simulink library "lib_FOWLTY"  (R2022a)
settings: Solver=ode45  StartTime=0.0  StopTime=10.0  RelTol=1e-3  EnableMultiTasking=on
undefined symbols (not defined in the file or in its folder): sigbuilder_block, tMax, wind
libraries: simulink x1
settings Model: Creator=grunnet  LastModifiedBy=Yerai
settings SolverCC: AlgebraicLoopSolver=TrustRegion
settings DataIOCC: LimitDataPoints=on  SaveFormat=Array  ReturnWorkspaceOutputs=off
settings OptimizationCC: ExpressionDepthLimit=2147483647  LifeSpan=inf
settings DebuggingCC: UnderspecifiedInitializationDetection=Classic  MergeDetectMultiDrivingBlocksExec=none  SolverPrmCheckMsg=warning  FcnCallInpInsideContextMsg=warning  UnconnectedInputMsg=warning  UnconnectedOutputMsg=warning  UnconnectedLineMsg=warning  StateNameClashWarn=warning  SFUnexpectedBacktrackingDiag=warning  SFNoUnconditionalDefaultTransitionDiag=warning  SFExecutionAtInitializationDiag=none  ArithmeticOperatorsInVariantConditions=warning
settings HardwareCC: ProdBitPerPointer=32  ProdBitPerSizeT=32  ProdBitPerPtrDiffT=32  ProdLargestAtomicFloat=None  ProdIntDivRoundTo=Undefined  ProdEndianess=Unspecified  ProdWordSize=32  ProdHWDeviceType=32-bit Generic
settings ModelReferenceCC: PropagateSignalLabelsOutOfModel=off
settings SFSimCC: SimUseLocalCustomCode=off  CustomCodeUndefinedFunction=UseInterfaceOnly
settings RTWCC: RTWUseLocalCustomCode=off  DLArmComputeVersion=19.05
settings CodeAppCC: StateflowObjectComments=on
settings GRTTargetCC: TargetLangStandard=C89/C90 (ANSI)  CombineOutputUpdateFcns=off  GRTInterface=on
settings ConfigComp: CovMetricSettings=dw  CovSaveCumulativeToWorkspaceVar=on  CovSaveSingleToWorkspaceVar=on  CovExternalEMLEnable=off

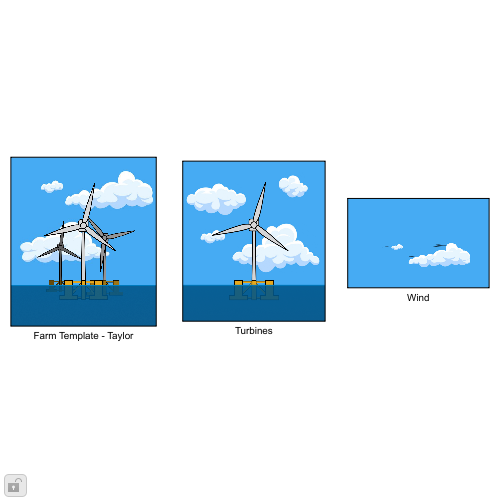
[thumbnail: Simulink's stored preview of the top-level diagram]
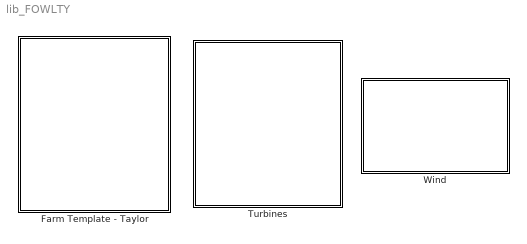
== system lib_FOWLTY ==
  Farm Template - Taylor : Subsystem  mask(Aeolus){}
      mask help: Wind Farm Template for the Aeolus Farm Simulator.
      settings: OpenFcn=create_windfarm()
      mask Display: image(imread(['FOWT_farm.png']))
  Turbines : Subsystem
      settings: OpenFcn=libturbines
      mask Display: image('FOWT.png')
  Wind : Subsystem
      settings: OpenFcn=libwind
      mask Display: image(imread('wind.png'))

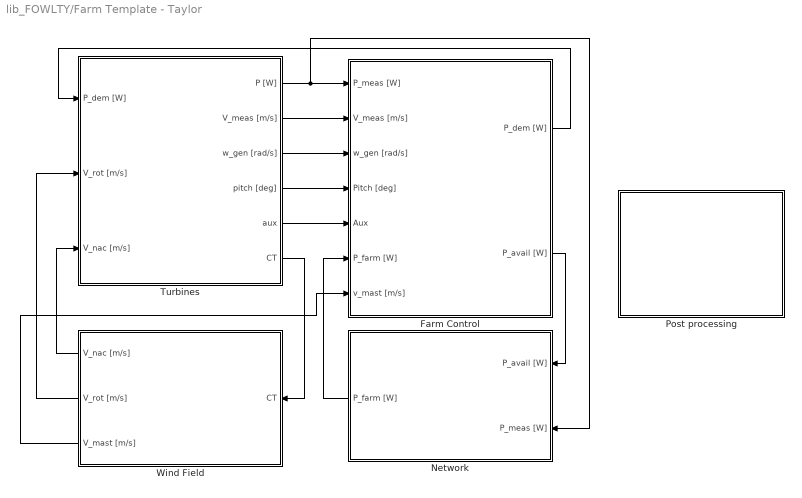
== system lib_FOWLTY/Farm Template - Taylor ==
  Farm Control : Subsystem  mask(Farm Control){Ts=5}
      mask prompts: Ts "Control Sample Time"
      mask help: A Farm controller with proportional distribution
      mask init:
      | parm=get_param(gcb,'UserData');
      | CTs=Ts;
      mask Display:
      | image('controller.png');
      | 
      | port_label('input',1,'P_meas [W]')
      | port_label('input',2,'V_meas [m/s]')
      | port_label('input',3,'w_gen [rad/s]')
      | port_label('input',4,'Pitch [deg]')
      | port_label('input',5,'Aux')
      | port_label('input',6,'P_farm_dem [W]')
      | port_label('input',7,'V_mast [m/s]')
      | 
      | 
      | port_label('output',1,'P_dem[W]')
      | port_label('output',2,'P_avail [W]')
  Network : Subsystem  mask{mode=Absolute, Ts=30, pref=12e6, rate=1e6, delta=2e6, db=.1, cb=1, maxp=15e6, minp=10e6, freq=50, delay=.1}
      mask prompts: mode "Operating Mode"; Ts "Sample Time [s]"; pref "Power reference [W]"; rate "Power rate limit [W/s]"; delta "Reserved power [W]"; db "Dead band [Hz]"; cb "Control band [Hz]"; maxp "Maximum power [W]"; minp "Minimum power [W]"; freq "Frequency reference [Hz]"; delay "Communication delay [s]"
      mask help: Network Operator Parameters
      mask init:
      | parm.Ts=Ts;
      | parm.mode=mode;
      | switch(mode)
      |     case 1
      |         parm.settings(1)=pref;
      |     case 2
      |         parm.settings(1)=delta;
      |     case 3
      |         parm.settings(1)=pref;
      |     case 4
      |         parm.settings(1)=rate;
      |     case 5
      |         parm.settings(1)=db;
      |         parm.settings(2)=cb;
      |         parm.settings(3)=maxp;
      |         parm.settings(4)=minp;
      |         parm.settings(5)=freq;
      |     otherwise
      |         parm.settings(1)=1e10;
      | end
      | parm.delay=delay;
      mask TypeOptions mode: Absolute | Delta | Balance | Rate Limit | Frequency
      mask Callback mode:
      | m=get_param(gcb,'mode');
      | switch(m)
      |     case 'Absolute'
      |         mv={'on','on','on','off','off', ...
      |             'off','off','off','off','off','on'};
      |     case 'Delta'
      |         mv={'on','on','off','off','on', ...
      |             'off','off','off','off','off','on'};
      |     case 'Balance'
      |         mv={'on','on','on','off','off', ...
      |             'off','off','off','off','off','on'};
      |     case 'Rate Limit'
      |         mv={'on','on','off','on','off', ...
      |             'off','off','off','off','off','on'};
      |     case 'Frequency'
      |         mv={'on','on','off','off','off', ...
      |             'on','on','on','on','on','on'};
      | end
      | 
      | set_param(gcb,'MaskVisibilities',mv);
      mask Display:
      | image('Network.png');
      | 
      | 
      | port_label('output',1,'P_farm_dem [W]')
      | port_label('input',1,'P_avail[W]')
      | port_label('input',2,'P_meas [W]')
  Post processing : Subsystem
      mask Display: image(imread('postproc.png'))
  Turbines : Subsystem  LoadFcn=|  mask(Data logging setup){mode=Wind Sync, ts=-1, dec=1}
      | p=get_param(gcb,'UserData');                                                                                                                                            
      | %If not compatible                                                                                                                                                      
      |                                                                                                                                                                         
      | %Check to avoid template warning                                                                                                                                        
      | if(~isempty(p))                                                                                                                                                         
      |                                                                                                                                                                         
      | 	if(~iscompat(p.version))                                                                                                                                               
      | 		warndlg('The version of SimWindFarm used to create this model does not match the installed version! This may result in undefined behaviour.','Model version mismatch')
      | 	end                                                                                                                                                                    
      | end
      mask prompts: mode "Sample Mode"; ts "Sample Time"; dec "Decimation"
      mask help: Adjust the amount of data logged from the turbines
      mask init:
      | switch(mode)
      |     case 3 % inherit
      |         TTs = -1;
      |     case 1 % Wind
      |         TTs = str2num(get_param([extractBefore(gcb,'/Turbines') '/Wind Field/CTrate'],'OutPortSampleTime'));
      |     case 2 % costum
      |         TTs = ts; 
      | end
      | 
      | assignin('base','SWFdecimation',dec);
      | assignin('base','SWFTTs',TTs);
      mask Help:
      | Wind Synch - Data is logged with the wind field time step
      | Specify - Set a custom sampling time
      | Inherit - Inherit from output port
      mask TypeOptions mode: Wind Sync | Specify | Inherit
      mask Display:
      | image('FOWT_farm.png')
      | 
      | 
      | port_label('input',1,'P_dem [W]')
      | port_label('input',2,'V_rot [m/s]')
      | port_label('input',3,'V_nac [m/s]')
      | %port_label('input',4,'Fex')
      | %port_label('input',5,'Fault signal')
      | port_label('output',1,'P [W]')
      | port_label('output',2,'v_meas [m/s]')
      | port_label('output',3,'w_gen [rad/s]')
      | port_label('output',4,'pitch [deg]')
      | port_label('output',5,'aux')
      | port_label('output',6,'CT')
  Wind Field : Subsystem
      settings: OpenFcn=|
      | [wfile,wpath,wfidx]=uigetfile('*.mat','Select a Wind Data File');
      | if isequal(wfile,0) || isequal(wpath,0)
      |    return
      | end
      | 
      | %Loads wind profile data
      | l=load([wpath wfile]);
      | p=get_param([gcb '/Ambient Field'],'UserData');
      | 
      | %Check compatible mean wind speed
      | if(~isfield(l.wind,'Umean') | ~isfield(p,'Umean'))
      |     warning('WarnTests:convertTest','Mean wind speed is not part of wind field struct.\n Consider updating model or windfield to newest version of SimWindFarm \n To get correct simulation behaviour, the mean wind speed of the wind field needs to be equal to the one used when farm model is created')
      | else
      |     if (~isequal(p.Umean,l.wind.Umean))
      |         str_wind_speeds = sprintf('Old mean wind speed (%d m/s) does not correspond to new mean wind speed (%d m/s). \n This may cause the simulation to be incorrect because wake delay between turbines changes. \n The solution is to create a new model with the desired average wind speed. \n Setting new windfield anyway.....', p.Umean, l.wind.Umean);
      |         warndlg(str_wind_speeds, 'Mean wind speed incompatibility')
      |     end
      | end
      | 
      | %Check for correct wind field type
      | if(isfield(l.wind,'ambient_wind'))
      |     errordlg('It is not the correct wind field type. Probably a no_taylor type wind field. See create_windfield()','Wind field invalid')
      |    return
      | end
      | 
      | %Check for compatible wind field
      | if (~isequal(p.grid,l.wind.grid))
      |     str_grids = sprintf('\n            Model     New wind \n size          %d         %d \n xsize       %d       %d \n ysize        %d      %d \n Try to type: help create_windfield',p.grid.size, l.wind.grid.size, p.grid.xsize, l.wind.grid.xsize, p.grid.ysize, l.wind.grid.ysize);
      |     errordlg(['The wind fields must have the same grid' str_grids],'Wind field Error')
      |    return
      | end
      | 
      | %If the wind field is too short, reset the simulation time
      | if(p.SimTime < eval(get_param(bdroot,'StopTime')))
      |     warndlg('The model simulation time is longer than windfield. Resetting model simulation time')
      |     set_param(bdroot,'StopTime',num2str(p.SimTime))
      | end
      | 
      | %Change wf sample time
      | set_param([gcb '/CTrate'],'OutPortSampleTime',num2str(l.wind.Ts))
      | 
      | %Add old turbine position data
      | l.wind.xgrids=p.xgrids;
      | 
      | %Save the new parameters
      | set_param([gcb '/Ambient Field'],'UserData',l.wind);
      mask Display:
      | image('Wind.png')
      | 
      | port_label('input',1,'CT')
      | 
      | port_label('output',1,'V_nac [m/s]')
      | port_label('output',2,'V_rot [m/s]')
      | port_label('output',3,'V_mast [m/s]')
  wires:
  Turbines/6(CT) -> Wind Field/1(CT)
  Wind Field/1(V_nac [m/s]) -> Turbines/3(V_nac [m/s])
  Wind Field/2(V_rot [m/s]) -> Turbines/2(V_rot [m/s])
  Farm Control/1(P_dem [W]) -> Turbines/1(P_dem [W])
  Turbines/2(V_meas [m/s]) -> Farm Control/2(V_meas [m/s])
  Turbines/1(P [W]) -> Network/2(P_meas [W]), Farm Control/1(P_meas [W])
  Farm Control/2(P_avail [W]) -> Network/1(P_avail [W])
  Network/1(P_farm [W]) -> Farm Control/6(P_farm [W])
  Turbines/5(aux) -> Farm Control/5(" Aux")
  Turbines/4(pitch [deg]) -> Farm Control/4(Pitch [deg])
  Turbines/3(w_gen [rad/s]) -> Farm Control/3(w_gen [rad/s])
  Wind Field/3(V_mast [m/s]) -> Farm Control/7(" v_mast [m/s]")

== system lib_FOWLTY/Turbines ==

== system lib_FOWLTY/Wind ==

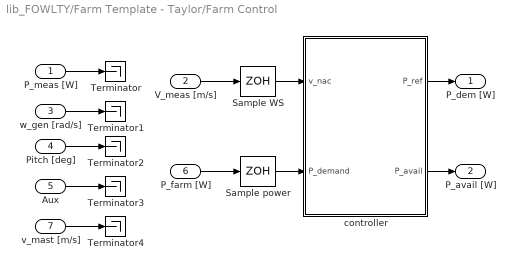
== system lib_FOWLTY/Farm Template - Taylor/Farm Control ==
  P_meas [W] : Inport
  V_meas [m/s] : Inport  Port=2
  w_gen [rad/s] : Inport  Port=3
  Pitch [deg] : Inport  Port=4
  " Aux" : Inport  Port=5
  P_farm [W] : Inport  Port=6
  " v_mast [m/s]" : Inport  Port=7
  Sample WS : ZeroOrderHold  SampleTime=wind.Ts
  Sample power : ZeroOrderHold  SampleTime=wind.Ts
  Terminator{,1..4} (5 alike) : Terminator
  controller : MATLAB Function  TreatAsAtomicUnit=on
  P_dem [W] : Outport
  P_avail [W] : Outport  Port=2
  wires:
  P_farm [W]/1 -> Sample power/1
  controller/1(P_ref) -> P_dem [W]/1
  controller/2(P_avail) -> P_avail [W]/1
  Sample power/1 -> controller/2(P_demand)
  V_meas [m/s]/1 -> Sample WS/1
  Sample WS/1 -> controller/1(v_nac)
  P_meas [W]/1 -> Terminator/1
  w_gen [rad/s]/1 -> Terminator1/1
  Pitch [deg]/1 -> Terminator2/1
  " Aux"/1 -> Terminator3/1
  " v_mast [m/s]"/1 -> Terminator4/1

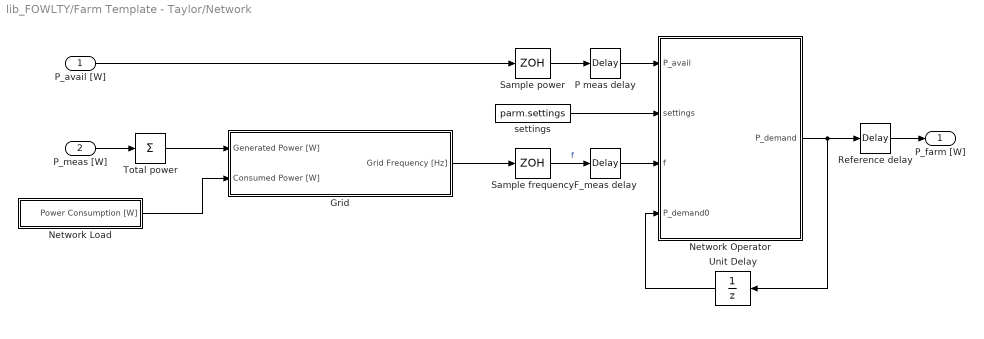
== system lib_FOWLTY/Farm Template - Taylor/Network ==
  P_avail [W] : Inport
  P_meas [W] : Inport  Port=2
  F_meas delay : TransportDelay  DelayTime=parm.delay
  Grid : Subsystem  mask{fgain=2e-9}
      mask prompts: fgain "Power to frequency gain"
      mask init:
      | frequencygain=fgain;
  Network Load : Subsystem  mask{maxp=15e6}
      mask prompts: maxp "Max farm power [W]"
      mask init:
      | maxpower=maxp;
  Network Operator : MATLAB Function  TreatAsAtomicUnit=on
  P meas delay : TransportDelay  DelayTime=parm.delay
  Reference delay : TransportDelay  DelayTime=.01
  Sample frequency : ZeroOrderHold  SampleTime=parm.Ts
  Sample power : ZeroOrderHold  SampleTime=wind.Ts
  Total power : Sum  Inputs=+
  Unit Delay : UnitDelay  SampleTime=wind.Ts  HasFrameUpgradeWarning=on
  settings : Constant  Value=parm.settings  OutDataTypeStr=double  SampleTime=wind.Ts
  P_farm [W] : Outport
  wires:
  Unit Delay/1 -> Network Operator/4(P_demand0)
  Sample frequency/1 -> F_meas delay/1  "f"
  settings/1 -> Network Operator/2(settings)
  Sample power/1 -> P meas delay/1
  P_avail [W]/1 -> Sample power/1
  Network Operator/1(P_demand) -> Unit Delay/1, Reference delay/1
  F_meas delay/1 -> Network Operator/3(f)
  P meas delay/1 -> Network Operator/1(P_avail)
  Reference delay/1 -> P_farm [W]/1
  Total power/1 -> Grid/1(Generated Power [W])
  Grid/1(Grid Frequency [Hz]) -> Sample frequency/1
  Network Load/1(Power Consumption [W]) -> Grid/2(Consumed Power [W])
  P_meas [W]/1 -> Total power/1

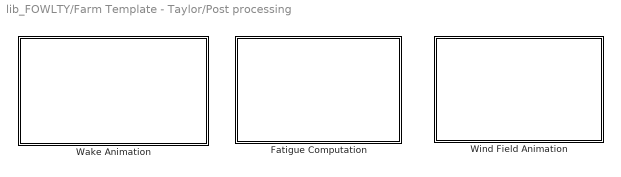
== system lib_FOWLTY/Farm Template - Taylor/Post processing ==
  Fatigue Computation : Subsystem
      settings: OpenFcn=fatigue=fatiguegui(logsout);
      mask Display: image(imread('rainflow.png'))
  Wake Animation : Subsystem
      settings: OpenFcn=|
      | sys=bdroot(gcb);
      | create_wakeanim(sys,logsout);
      mask Display: image(imread('wakeanim.png'))
  Wind Field Animation : Subsystem
      settings: OpenFcn=|
      | sys=bdroot(gcb);
      | windanim(sys,logsout);
      mask Display: image(imread('windanim.png'))

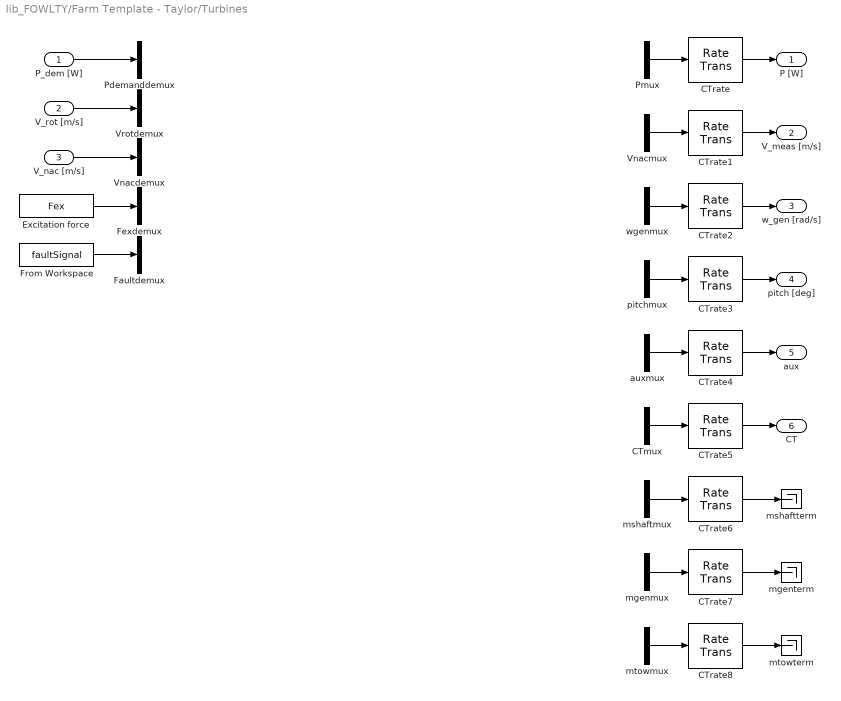
== system lib_FOWLTY/Farm Template - Taylor/Turbines ==
  P_dem [W] : Inport
  V_rot [m/s] : Inport  Port=2
  V_nac [m/s] : Inport  Port=3
  CTmux : Mux  Inputs=2
  CTrate{,1..8} (9 alike) : RateTransition  Deterministic=off  OutPortSampleTime=wind.Ts
  Excitation force : FromWorkspace  VariableName=Fex
  Faultdemux : Demux  Outputs=3
  Fexdemux : Demux  Outputs=3
  From Workspace : FromWorkspace  VariableName=faultSignal
  Pdemanddemux : Demux  Outputs=3
  Pmux : Mux  Inputs=2
  Vnacdemux : Demux  Outputs=3
  Vnacmux : Mux  Inputs=2
  Vrotdemux : Demux  Outputs=3
  auxmux : Mux  Inputs=2
  mgenmux : Mux  Inputs=2
  mgenterm : Terminator
  mshaftmux : Mux  Inputs=2
  mshaftterm : Terminator
  mtowmux : Mux  Inputs=2
  mtowterm : Terminator
  pitchmux : Mux  Inputs=2
  wgenmux : Mux  Inputs=2
  P [W] : Outport
  V_meas [m/s] : Outport  Port=2
  w_gen [rad/s] : Outport  Port=3
  pitch [deg] : Outport  Port=4
  aux : Outport  Port=5
  CT : Outport  Port=6
  wires:
  V_nac [m/s]/1 -> Vnacdemux/1
  P_dem [W]/1 -> Pdemanddemux/1
  V_rot [m/s]/1 -> Vrotdemux/1
  Pmux/1 -> CTrate/1
  CTmux/1 -> CTrate5/1
  Vnacmux/1 -> CTrate1/1
  pitchmux/1 -> CTrate3/1
  auxmux/1 -> CTrate4/1
  wgenmux/1 -> CTrate2/1
  mshaftmux/1 -> CTrate6/1
  mtowmux/1 -> CTrate8/1
  CTrate/1 -> P [W]/1
  CTrate1/1 -> V_meas [m/s]/1
  CTrate2/1 -> w_gen [rad/s]/1
  CTrate3/1 -> pitch [deg]/1
  CTrate4/1 -> aux/1
  CTrate5/1 -> CT/1
  CTrate6/1 -> mshaftterm/1
  CTrate8/1 -> mtowterm/1
  Excitation force/1 -> Fexdemux/1
  From Workspace/1 -> Faultdemux/1
  CTrate7/1 -> mgenterm/1
  mgenmux/1 -> CTrate7/1

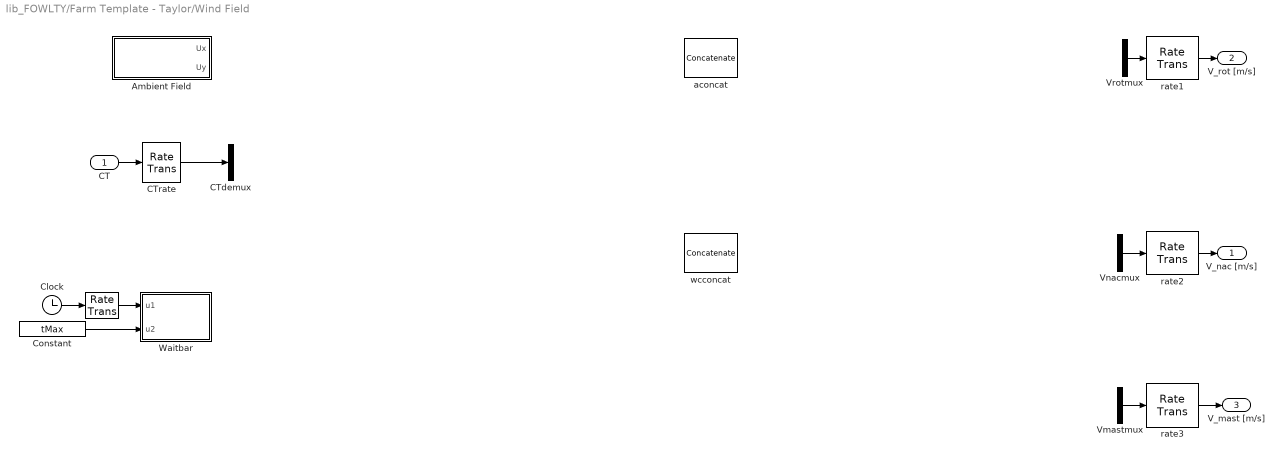
== system lib_FOWLTY/Farm Template - Taylor/Wind Field ==
  CT : Inport
  " " : RateTransition  Deterministic=off  OutPortSampleTime=wind.Ts
  Ambient Field : Subsystem
      mask init:
      | wind=get_param(gcb,'UserData');
  CTdemux : Demux  Outputs=3
  CTrate : RateTransition  Deterministic=off  OutPortSampleTime=wind.Ts
  Clock : Clock
  Constant : Constant  Value=tMax  SampleTime=100*wind.Ts
  Vmastmux : Mux  Inputs=2
  Vnacmux : Mux  Inputs=2
  Vrotmux : Mux  Inputs=2
  Waitbar : MATLAB Function  TreatAsAtomicUnit=on
  aconcat : Concatenate  Mode=Multidimensional array  ConcatenateDimension=2
  rate1 : RateTransition  Deterministic=off  OutPortSampleTime=wind.Ts
  rate2 : RateTransition  Deterministic=off  OutPortSampleTime=wind.Ts
  rate3 : RateTransition  Deterministic=off  OutPortSampleTime=wind.Ts
  wcconcat : Concatenate  Mode=Multidimensional array  ConcatenateDimension=2
  V_nac [m/s] : Outport
  V_rot [m/s] : Outport  Port=2
  V_mast [m/s] : Outport  Port=3
  wires:
  CT/1 -> CTrate/1
  Vrotmux/1 -> rate1/1
  Vnacmux/1 -> rate2/1
  CTrate/1 -> CTdemux/1
  rate1/1 -> V_rot [m/s]/1
  rate2/1 -> V_nac [m/s]/1
  Vmastmux/1 -> rate3/1
  rate3/1 -> V_mast [m/s]/1
  Constant/1 -> Waitbar/2(u2)
  " "/1 -> Waitbar/1(u1)
  Clock/1 -> " "/1

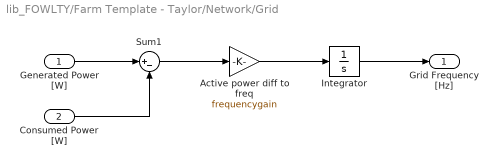
== system lib_FOWLTY/Farm Template - Taylor/Network/Grid ==
  Generated Power [W] : Inport
  Consumed Power [W] : Inport  Port=2
  Active power diff to freq : Gain  Gain=frequencygain
  Integrator : Integrator  InitialCondition=50  LimitOutput=on  UpperSaturationLimit=100  LowerSaturationLimit=0
  Sum1 : Sum  Inputs=|+-
  Grid Frequency [Hz] : Outport
  wires:
  Integrator/1 -> Grid Frequency [Hz]/1
  Sum1/1 -> Active power diff to freq/1
  Active power diff to freq/1 -> Integrator/1
  Generated Power [W]/1 -> Sum1/1
  Consumed Power [W]/1 -> Sum1/2

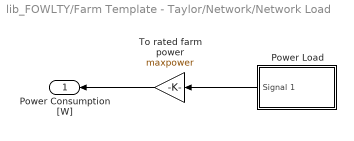
== system lib_FOWLTY/Farm Template - Taylor/Network/Network Load ==
  Power Load : Subsystem  Tag=STV Subsys  LoadFcn=sigbuilder_block('load');  StartFcn=sigbuilder_block('start');  StopFcn=sigbuilder_block('stop');  ClipboardFcn=sigbuilder_block('clipboard');  mask(Sigbuilder block){tuvar=[0:10]}
      mask help: Sigbuilder GUI
      mask init:
      | if ~strcmp(get_param(bdroot(gcbh),'SimulationStatus'),'stopped') tuvar = sigbuilder_block('maskInit'); end
      settings: CopyFcn=sigbuilder_block('copy');  DeleteFcn=sigbuilder_block('delete');  ModelCloseFcn=sigbuilder_block('modelClose');  PreSaveFcn=sigbuilder_block('preSave');  PauseFcn=sigbuilder_block('pause')  ContinueFcn=sigbuilder_block('continue')  NameChangeFcn=sigbuilder_block('namechange');  OpenFcn=sigbuilder_block('open',[437.6 199.2 550.4 400 ]);  CloseFcn=sigbuilder_block('close');
      mask Display: plot(0, 0, 100, 100,[2, 2, 32, 32, 2], [68, 8, 8, 68, 68],[32, 2], [38, 38], [32, 19, 2],[53, 60, 44], [32, 17, 17, 2],[16, 16, 31, 31]);txt = getActiveGroup(gcbh);text(2, 100, txt,'verticalAlignment', 'top');
  To rated farm power : Gain  Gain=maxpower
  Power Consumption [W] : Outport
  wires:
  Power Load/1(Signal 1) -> To rated farm power/1
  To rated farm power/1 -> Power Consumption [W]/1

== system lib_FOWLTY/Farm Template - Taylor/Post processing/Fatigue Computation ==

== system lib_FOWLTY/Farm Template - Taylor/Post processing/Wake Animation ==

== system lib_FOWLTY/Farm Template - Taylor/Post processing/Wind Field Animation ==

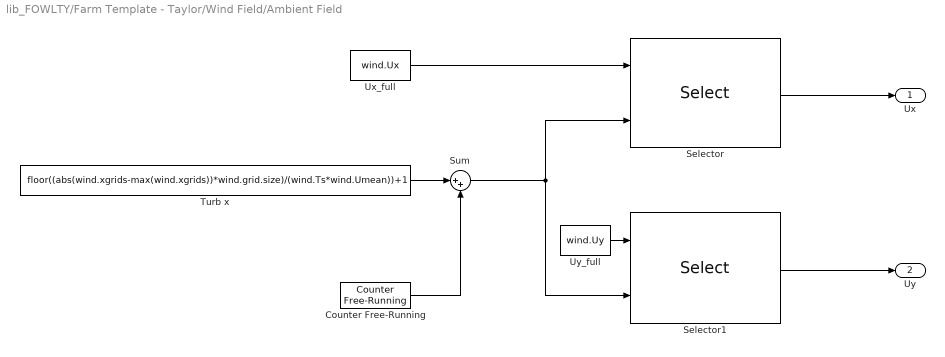
== system lib_FOWLTY/Farm Template - Taylor/Wind Field/Ambient Field ==
  Counter Free-Running : simulink/Sources/Counter Free-Running  NumBits=32  tsamp=wind.Ts
  Selector : Selector  NumberOfDimensions=2  InputPortWidth=3  IndexOptions=Select all,Index vector (port)  Indices=[1 3],1  OutputSizes=1,1
  Selector1 : Selector  NumberOfDimensions=2  InputPortWidth=3  IndexOptions=Select all,Index vector (port)  Indices=[1 3],1  OutputSizes=1,1
  Sum : Sum  Inputs=|++
  Turb x : Constant  Value=floor((abs(wind.xgrids-max(wind.xgrids))*wind.grid.size)/(wind.Ts*wind.Umean))+1
  Ux_full : Constant  Value=wind.Ux
  Uy_full : Constant  Value=wind.Uy
  Ux : Outport
  Uy : Outport  Port=2
  wires:
  Selector/1 -> Ux/1
  Selector1/1 -> Uy/1
  Turb x/1 -> Sum/1
  Counter Free-Running/1 -> Sum/2
  Sum/1 -> Selector/2, Selector1/2
  Uy_full/1 -> Selector1/1
  Ux_full/1 -> Selector/1

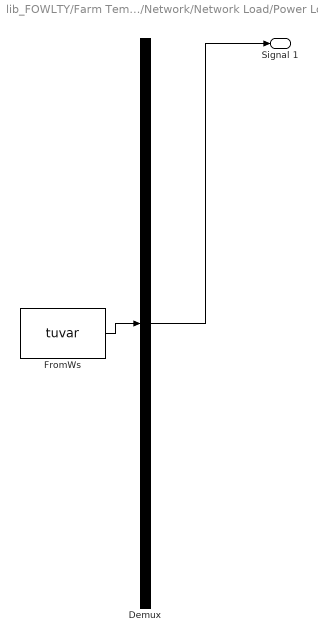
== system lib_FOWLTY/Farm Template - Taylor/Network/Network Load/Power Load ==
  Demux : Demux  Tag=STV Demux  Outputs=1
      settings: DisplayOption=none
  FromWs : FromWorkspace  Tag=STV FromWs  VariableName=tuvar
      SigBuilderData=|
      | common.afterFinalStr = 'Extrapolate'
      | common.sampleTime = 0
      | dataSet.timeRange = [0 1000]
      | dataSet.name = 'Group 1'
      | sbobj.Groups.Name = 'Group 1'
      | sbobj.Groups.Signals.Name = 'Signal 1'
      | sbobj.Groups.Signals.XData = [0 25 100 200 500 1000]
      | sbobj.Groups.Signals.YData = [0.1 0.1 0.7 0.7 0.9 0.85]
  Signal 1 : Outport  Tag=STV Outport
  wires:
  Demux/1 -> Signal 1/1
  FromWs/1 -> Demux/1

== matlab function lib_FOWLTY/Farm Template - Taylor/Wind Field/Waitbar ==
  data: u1 input; u2 input
function fcn(u1,u2)
coder.extrinsic('waitbar');

wb = waitbar(u1/u2);

if (u1/u2) == 1
    close(wb)
end

== matlab function lib_FOWLTY/Farm Template - Taylor/Farm Control/controller ==
  data: v_nac input; P_demand input; parm parameter; P_ref output; P_avail output
function [P_ref,P_avail]  = Farm_Controller(v_nac,P_demand,parm)
%
% Farm_Controller estimates the available power at the farm and distributes the 
% power references proportional to the available power at each wind turbine.
%
% [P_ref,P_avail_total]  = Farm_Controller(v_nac,P_demand)
%
% vn : the wind speed at wind turbine number n.
%
% P_demand : The demanded power by the operator.
%
% P_ref : The power reference for the wind turbines.
%
% P_avail : Available power at the farm level
%
%
% Version 1: 2009-04-10 sms
% Version 2: 2009-12-04 grunnet
% By : S. Mohsen N. Soltani & Jacob D. Grunnet
% Aalborg University, Dept. of Electronic Systems, Section of Automation
% and Control
% E-mail: sms@es.aau.dk
% E-mail: grunnet@es.aau.dk

rho=parm.rho; %air dencity
R=parm.radius; %rotor radius
rated=parm.rated; %Rated power
N=parm.N; %Number of turbines
Cp=parm.Cp; % Max cp of the turbines

P_a=zeros(N,1);
P_ref=zeros(N,1);

% Compute available power at each turbine
for i=1:N
    %P_a=1/2*pi*r^2*Cp*v^3
    P_a(i)=min(rated(i),(pi/2)*rho*R(i)^2*v_nac(i)^3*Cp(i));
end

%Compute total available power
P_avail=sum(P_a);

%Distribute power according to availibility
for i=1:N
    P_ref(i)=max(0,min(rated(i),P_demand*P_a(i)/P_avail));
end

== matlab function lib_FOWLTY/Farm Template - Taylor/Network/Network Operator ==
  data: P_avail input; settings input; f input; P_demand output; P_demand0 input; parm parameter
function P_demand = TSO(P_avail,settings,f,P_demand0,parm)
%
% TSO provides the demanded power to the wind farm controller.
%
% P_avail : Aavailable power at the farm level.
%
% mode : The operation mode.
%
% settings : The settings corresponding to the operational mode
%
% f : Frequency of the network
%
% P_deamnd0 : The last update of the deamded power
%
% Ts : Sample Time
%
% Time-stamp: <2009-04-10 sms>
% Version 1: 2009-04-10 sms 
% By : S. Mohsen N. Soltani
% Aalborg University, Dept. of Electronic Systems, Section of Automation
% and Control
% E-mail: sms@es.aau.dk
% 
 P=0;
 switch(parm.mode)
     case 1 %Absolute active power control
        P=settings(1);
%       % type='Full power';
     case 2 %Delta mode
        P=P_avail-settings(1);
%       % type='Delta mode';
     case 3 %Balance
        P=settings(1);
%       % type='Balance';
     case 4 %Rate limiter
        P=min(P_avail,settings(1)*parm.Ts+P_demand0);
%       % type='Rate limiter';
     case 5 %Frequency Control
        deadb=settings(1);
        contb=settings(2);
        maxp=settings(3);
        minp=settings(4);
        f=f-settings(5); % To provide Delta f
        if ( f<= deadb && f>=-deadb)
            P=0.5*(maxp+minp);
        elseif f>= contb
            P=minp;
        elseif f<= -contb
            P=maxp;
        elseif ( f>deadb && f<contb)
            P=0.5*(maxp+minp)-0.5*(maxp-minp)*(f-deadb)/(contb-deadb);
        elseif ( f<-deadb && f>-contb)
            P=0.5*(maxp+minp)-0.5*(maxp-minp)*(f+deadb)/(contb-deadb);
        end
%       % type='Frequency Control';
     otherwise %Unknown
        P=P_avail;
%       % type='Unknown Mode';
 end
%        

P_demand=max(0,P);
